simulink model "inverted_linear_pendulum"  (R2025b)
settings: Solver=VariableStepAuto  StartTime=0.0  StopTime=10  RelTol=1e-3
values from neighbouring files (symbols this model uses):
  Ae = [[Anum P ... (first row only)    [linear_pendulum.m]
  Anum = double(subs(A, [M m l g], [M_val m_val l_val g_val]))    [linear_pendulum.m]
  Be = [Bnum; zeros(3,2)]    [linear_pendulum.m]
  Bnum = double(subs(B, [M m l g], [M_val m_val l_val g_val]))    [linear_pendulum.m]
  Ce = [Cnum -Q]    [linear_pendulum.m]
  Cnum = C    [linear_pendulum.m]
  Gamma_sol = reshape(vals(n*r+1:end), m, r)    [solver_regEquations.m]
  K = place(Anum, Bnum, poles_K)    [linear_pendulum.m]
  Le = place(Ae', Ce', poles_obs_e)'    [linear_pendulum.m]
  Pi_sol = reshape(vals(1:n*r), n, r)    [solver_regEquations.m]
  Q = [1 0 0 ... (first row only)    [linear_pendulum.m]
  S = [0 4 0 ... (first row only)    [linear_pendulum.m]
settings Model: Creator=Armando  LastModifiedBy=Armando

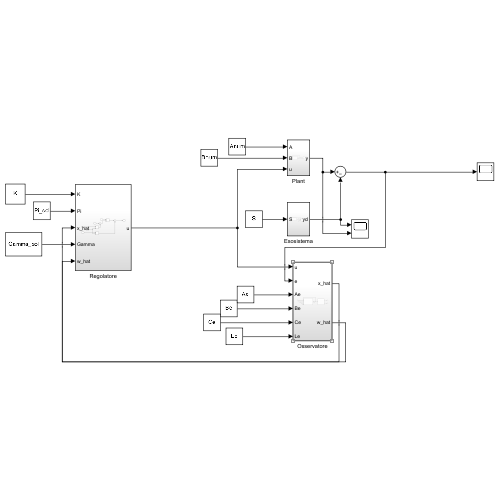
[thumbnail: Simulink's stored preview of the top-level diagram]
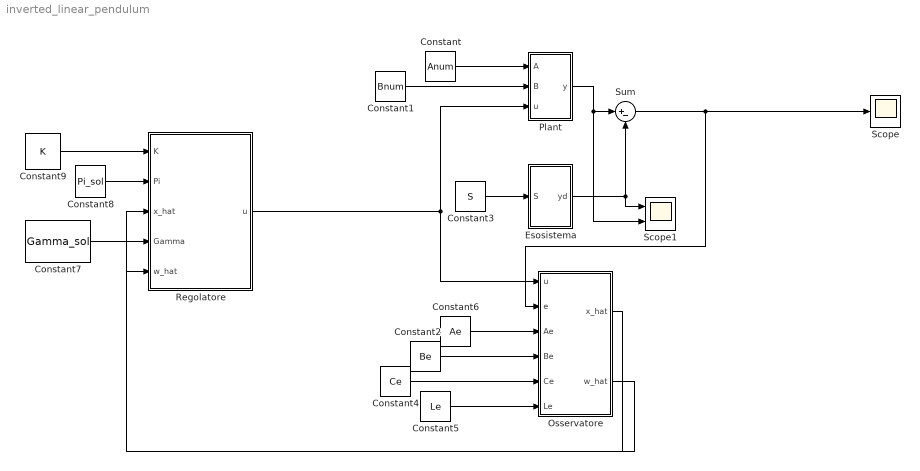
== system inverted_linear_pendulum ==
  Constant : Constant  Value=Anum
  Constant1 : Constant  Value=Bnum
  Constant2 : Constant  Value=Be
  Constant3 : Constant  Value=S
  Constant4 : Constant  Value=Ce
  Constant5 : Constant  Value=Le
  Constant6 : Constant  Value=Ae
  Constant7 : Constant  Value=Gamma_sol
  Constant8 : Constant  Value=Pi_sol
  Constant9 : Constant  Value=K
  Esosistema : Subsystem
  Osservatore : Subsystem
  Plant : Subsystem
  Regolatore : Subsystem
  Scope : Scope
      settings: ActiveDisplayYMinimum=-5.9595598814630142  ActiveDisplayYMaximum=23.636038933167132
  Scope1 : Scope  NumInputPorts=2
      settings: ActiveDisplayYMinimum=-2.2567198382375988  ActiveDisplayYMaximum=28.418609979183344
  Sum : Sum  Inputs=|+-
  wires:
  Constant/1 -> Plant/1(A)
  Constant1/1 -> Plant/2(B)
  Constant3/1 -> Esosistema/1(S)
  Plant/1(y) -> Scope1/2, Sum/1
  Esosistema/1(yd) -> Scope1/1, Sum/2
  Sum/1 -> Osservatore/2(e), Scope/1
  Constant6/1 -> Osservatore/3(Ae)
  Constant2/1 -> Osservatore/4(Be)
  Constant4/1 -> Osservatore/5(Ce)
  Constant5/1 -> Osservatore/6(Le)
  Regolatore/1(u) -> Plant/3(u), Osservatore/1(u)
  Constant9/1 -> Regolatore/1(K)
  Constant8/1 -> Regolatore/2(Pi)
  Osservatore/1(x_hat) -> Regolatore/3(x_hat)
  Constant7/1 -> Regolatore/4(Gamma)
  Osservatore/2(w_hat) -> Regolatore/5(w_hat)

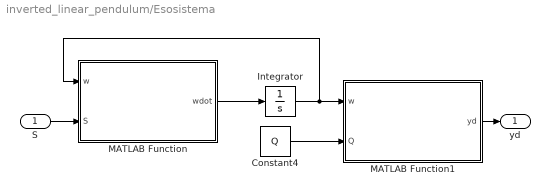
== system inverted_linear_pendulum/Esosistema ==
  S : Inport
  Constant4 : Constant  Value=Q
  Integrator : Integrator  InitialCondition=[1;0;3]
  MATLAB Function : MATLAB Function  TreatAsAtomicUnit=on
  MATLAB Function1 : MATLAB Function  TreatAsAtomicUnit=on
  yd : Outport
  wires:
  MATLAB Function/1(wdot) -> Integrator/1
  Integrator/1 -> MATLAB Function/1(w), MATLAB Function1/1(w)
  Constant4/1 -> MATLAB Function1/2(Q)
  MATLAB Function1/1(yd) -> yd/1
  S/1 -> MATLAB Function/2(S)

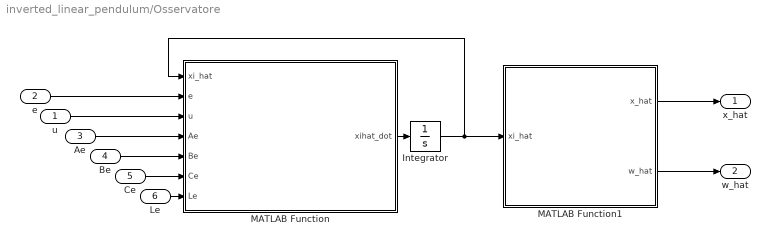
== system inverted_linear_pendulum/Osservatore ==
  u : Inport
  e : Inport  Port=2
  Ae : Inport  Port=3
  Be : Inport  Port=4
  Ce : Inport  Port=5
  Le : Inport  Port=6
  Integrator : Integrator  InitialCondition=[0;0;0;0;0;0;0]
  MATLAB Function : MATLAB Function  TreatAsAtomicUnit=on
  MATLAB Function1 : MATLAB Function  TreatAsAtomicUnit=on
  x_hat : Outport
  w_hat : Outport  Port=2
  wires:
  Ce/1 -> MATLAB Function/6(Ce)
  MATLAB Function1/1(x_hat) -> x_hat/1
  MATLAB Function/1(xihat_dot) -> Integrator/1
  Ae/1 -> MATLAB Function/4(Ae)
  Integrator/1 -> MATLAB Function/1(xi_hat), MATLAB Function1/1(xi_hat)
  Be/1 -> MATLAB Function/5(Be)
  Le/1 -> MATLAB Function/7(Le)
  u/1 -> MATLAB Function/3(u)
  MATLAB Function1/2(w_hat) -> w_hat/1
  e/1 -> MATLAB Function/2(e)

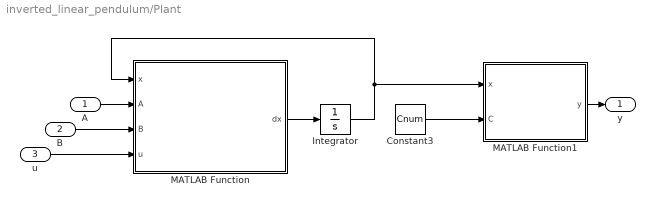
== system inverted_linear_pendulum/Plant ==
  A : Inport
  B : Inport  Port=2
  u : Inport  Port=3
  Constant3 : Constant  Value=Cnum
  Integrator : Integrator  InitialCondition=[0.1;0;0;1]
  MATLAB Function : MATLAB Function  TreatAsAtomicUnit=on
  MATLAB Function1 : MATLAB Function  TreatAsAtomicUnit=on
  y : Outport
  wires:
  B/1 -> MATLAB Function/3(B)
  MATLAB Function/1(dx) -> Integrator/1
  Constant3/1 -> MATLAB Function1/2(C)
  Integrator/1 -> MATLAB Function1/1(x), MATLAB Function/1(x)
  A/1 -> MATLAB Function/2(A)
  u/1 -> MATLAB Function/4(u)
  MATLAB Function1/1(y) -> y/1

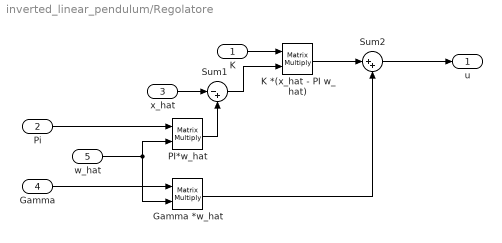
== system inverted_linear_pendulum/Regolatore ==
  K : Inport
  Pi : Inport  Port=2
  x_hat : Inport  Port=3
  Gamma : Inport  Port=4
  w_hat : Inport  Port=5
  Gamma *w_hat : Product  Multiplication=Matrix(*)
  K *(x_hat - PI w_hat) : Product  Multiplication=Matrix(*)
  PI*w_hat : Product  Multiplication=Matrix(*)
  Sum1 : Sum  Inputs=|-+
  Sum2 : Sum  Inputs=|++
  u : Outport
  wires:
  Gamma *w_hat/1 -> Sum2/2
  Sum1/1 -> K *(x_hat - PI w_hat)/2
  PI*w_hat/1 -> Sum1/2
  w_hat/1 -> Gamma *w_hat/2, PI*w_hat/2
  x_hat/1 -> Sum1/1
  K *(x_hat - PI w_hat)/1 -> Sum2/1
  Pi/1 -> PI*w_hat/1
  Sum2/1 -> u/1
  K/1 -> K *(x_hat - PI w_hat)/1
  Gamma/1 -> Gamma *w_hat/1

== matlab function inverted_linear_pendulum/Plant/MATLAB Function1 ==
  data: x input; y output; C input
function y = SystemOutput(x,C)
y = C*x;

== matlab function inverted_linear_pendulum/Plant/MATLAB Function ==
  data: x input; A input; B input; u input; dx output
function dx = SystemState(x,A,B,u)
dx = A*x + B*u;

== matlab function inverted_linear_pendulum/Esosistema/MATLAB Function ==
  data: w input; S input; wdot output
function wdot = Esosistema_state(w,S)
wdot = S*w;

== matlab function inverted_linear_pendulum/Esosistema/MATLAB Function1 ==
  data: w input; Q input; yd output
function yd = ydReconstruction(w,Q)
yd = Q*w;

== matlab function inverted_linear_pendulum/Osservatore/MATLAB Function ==
  data: xi_hat input; e input; u input; xihat_dot output; Ae input; Be input; Ce input; Le input
function xihat_dot = Osservatore(xi_hat,e,u,Ae,Be,Ce,Le)

xihat_dot= Ae * xi_hat + Be * u + Le*(e - (Ce*xi_hat)) ;

== matlab function inverted_linear_pendulum/Osservatore/MATLAB Function1 ==
  data: xi_hat input; x_hat output; w_hat output
function [x_hat, w_hat] = Separator(xi_hat)

x_hat = xi_hat(1:4);
w_hat = xi_hat(5:7);
end
